simulink model "tutorial_switched_nets"  (R2020a)
settings: Solver=FixedStepAuto  StartTime=0.0  StopTime=options.T_train  FixedStep=options.dt  MaxStep=.2  RelTol=1e-3
model workspace (MAT data in the model file):
  PID_TRESH = 0.3
undefined symbols (not defined in the file or in its folder): DiscIntNeverNeededParam, options
libraries: neural x72, simulink x2
(part 3 of 3)

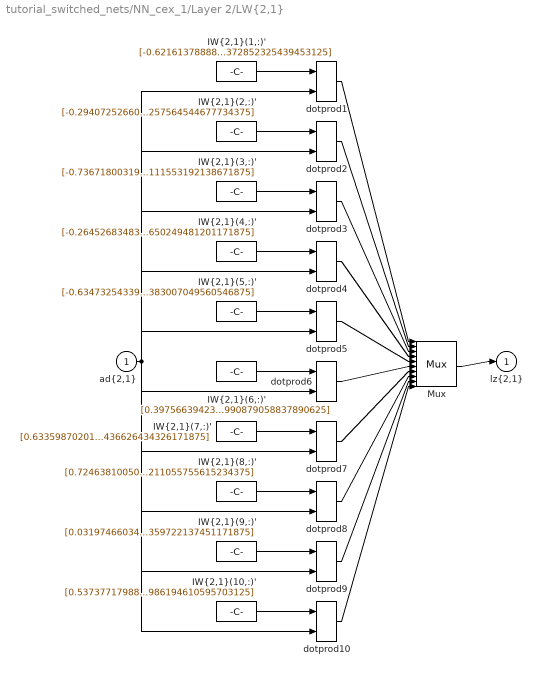
== system tutorial_switched_nets/NN_cex_1/Layer 2/LW{2,1} ==
  "ad{2,1}" : Inport  PortDimensions=20
      mask Display: e = 0.06;c1 = [120 230 180]/255;c2 = ([120 230 180]+0)/(256+128);c3 = ([120 230 180]+128)/(256+128);patch([0 1 1 0],[0 0 1 1],c1);patch([0 1 1 1-e 1-e 0+e],[0 0 1 1-e 0+e 0+e],c2);patch([0 0 1 1-e 0+e 0+e],[0 1 1 1-e 1-e 0+e],c3);plot([0 1 1 0 0],[0 0 1 1 0]);
  "IW{2,1}(1,:)'" : Constant  Value=[-0.62161378888258445041259392382926307618618011474609375;0.6148140198052960414543122169561684131622314453125;0.2096842513607183600132799483617418445646762847900390625;1.42295581141193760998930883943103253841400146484375;0.048162932797590825295674932249312405474483966827392578125;-0.329960676951758291597371908210334368050098419189453125;-0.243824039590348651262985413268324919044971466064453125;1.3156362099355323191929301174241118133068084716796875;0.65903370153445306467432374120107851922512054443359375;-0.1513918664553025872354652392459684051573276519775390625;-0.276008888794093854013311784001416526734828948974609375;0.476624595374437076689133618856430985033512115478515625;-0.7156998438142954110929849775857292115688323974609375;-0.350604636353502474577226166729815304279327392578125;0.359070507579784592433469470051932148635387420654296875;-0.088593367865525907145496375960647128522396087646484375;0.1682563802502727579035735061552259139716625213623046875;-0.157656333921617652915614371522678993642330169677734375;-0.082841065900426891221997038883273489773273468017578125;0.27502807794997086165977862037834711372852325439453125]
      mask Display: e = 0.06;c1 = [120 150 230]/255;c2 = ([120 150 230]+0)/383;c3 = ([120 150 230]+128)/383;patch([0 1 1 0],[0 0 1 1],c1);patch([0 1 1 1-e 1-e 0+e],[0 0 1 1-e 0+e 0+e],c2);patch([0 0 1 1-e 0+e 0+e],[0 1 1 1-e 1-e 0+e],c3);plot([0 1 1 0 0],[0 0 1 1 0]);disp('weights');
  "IW{2,1}(10,:)'" : Constant  Value=[0.53737717988913347166857192860334180295467376708984375;-0.54494791628668937111257264405139721930027008056640625;-0.327865563770393053655283210900961421430110931396484375;-0.2431502509493463082268505104366340674459934234619140625;-0.5506763502515099606426929312874563038349151611328125;0.2489329212039713412618624488459317944943904876708984375;0.2987323473001877172094964407733641564846038818359375;-0.37860104355034407408453489551902748644351959228515625;-0.523585007940606583787257477524690330028533935546875;0.25019101968781154443632885886472649872303009033203125;1.466831577856468005194301440496928989887237548828125;-0.68566639556574349168016624389565549790859222412109375;-0.51939265556673752666227983354474417865276336669921875;0.41255958958065652719682248061872087419033050537109375;-0.031873003307670851047550542034514364786446094512939453125;0.2298586870540712256971715987674542702734470367431640625;-0.2395025987128011346616318633095943368971347808837890625;0.39020251935073113624952156897052191197872161865234375;-0.14742684095521407794393553558620624244213104248046875;0.07941988847293768305490857528639025986194610595703125]
      mask Display: e = 0.06;c1 = [120 150 230]/255;c2 = ([120 150 230]+0)/383;c3 = ([120 150 230]+128)/383;patch([0 1 1 0],[0 0 1 1],c1);patch([0 1 1 1-e 1-e 0+e],[0 0 1 1-e 0+e 0+e],c2);patch([0 0 1 1-e 0+e 0+e],[0 1 1 1-e 1-e 0+e],c3);plot([0 1 1 0 0],[0 0 1 1 0]);disp('weights');
  "IW{2,1}(2,:)'" : Constant  Value=[-0.294072526609415518805690226145088672637939453125;1.524795289433424017033757991157472133636474609375;-0.11998592442710477590228634880986646749079227447509765625;0.88642225740235691677781915132072754204273223876953125;-1.13736511663246897541057478520087897777557373046875;0.56518577870423569731173074615071527659893035888671875;0.09829027065135671759055213669853401370346546173095703125;-1.0125569421073750131512269945233128964900970458984375;0.0165551729351459502026511216854487429372966289520263671875;0.82845463609548108951941003397223539650440216064453125;-0.9414506586527846554446341542643494904041290283203125;0.53562549536417181084146932334988377988338470458984375;-0.313691347770849782161661778445704840123653411865234375;0.47191275297145118816644071557675488293170928955078125;1.51617522055314868367759117973037064075469970703125;0.052764919032685243804881025653230608440935611724853515625;0.62185887535271133774728014032007195055484771728515625;0.0857756082959333643334076668907073326408863067626953125;0.25939285840393011550730761882732622325420379638671875;-0.224432553872412565709737464203499257564544677734375]
      mask Display: e = 0.06;c1 = [120 150 230]/255;c2 = ([120 150 230]+0)/383;c3 = ([120 150 230]+128)/383;patch([0 1 1 0],[0 0 1 1],c1);patch([0 1 1 1-e 1-e 0+e],[0 0 1 1-e 0+e 0+e],c2);patch([0 0 1 1-e 0+e 0+e],[0 1 1 1-e 1-e 0+e],c3);plot([0 1 1 0 0],[0 0 1 1 0]);disp('weights');
  "IW{2,1}(3,:)'" : Constant  Value=[-0.73671800319088820430124542326666414737701416015625;1.421314356877808382506600537453778088092803955078125;0.070753772050939911508748991764150559902191162109375;-0.56739678343006849647878198084072209894657135009765625;-0.85295856204789932686338715939200483262538909912109375;0.7386337240152494043599062933935783803462982177734375;0.0204718154347354776290135447425200254656374454498291015625;0.339184882494136863417821814437047578394412994384765625;-0.1881317420062826872850791914970614016056060791015625;-0.1339003061967665442200114966908586211502552032470703125;0.2394330914749966121579660693896585144102573394775390625;-0.6122315165013672011440348796895705163478851318359375;0.73620305612605718703633783661643974483013153076171875;0.38056001767816283187784165420453064143657684326171875;-0.1553003163997090096959396987585932947695255279541015625;0.0002292365914646561815548597706992950406856834888458251953125;0.0302889066986190315378113524502623477019369602203369140625;0.83805910127735006032168030287721194326877593994140625;0.1416795809112300352783364587594405747950077056884765625;-0.2543836837861146449313309858553111553192138671875]
      mask Display: e = 0.06;c1 = [120 150 230]/255;c2 = ([120 150 230]+0)/383;c3 = ([120 150 230]+128)/383;patch([0 1 1 0],[0 0 1 1],c1);patch([0 1 1 1-e 1-e 0+e],[0 0 1 1-e 0+e 0+e],c2);patch([0 0 1 1-e 0+e 0+e],[0 1 1 1-e 1-e 0+e],c3);plot([0 1 1 0 0],[0 0 1 1 0]);disp('weights');
  "IW{2,1}(4,:)'" : Constant  Value=[-0.264526834830059731640261588836438022553920745849609375;-0.84727523852972475015832287681405432522296905517578125;-0.443267493586528671389856981477350927889347076416015625;0.2034088335481475662280814731275313533842563629150390625;0.1795179798836086526581112821077113039791584014892578125;0.315091185795663253355058941451716236770153045654296875;-0.26441621089079669904009506353759206831455230712890625;0.167220214629539842832173235365189611911773681640625;0.4563687033643990531572853797115385532379150390625;0.49015080532649968336755819109384901821613311767578125;-0.554760108665810935946183235500939190387725830078125;1.386615644304538097486556580406613647937774658203125;-1.1832183710485491001662694543483667075634002685546875;-0.43202725012682130500962784935836680233478546142578125;-0.0781915813170765972017761669121682643890380859375;0.3670003065691587185170874363393522799015045166015625;-0.53144904234001433263046010324615053832530975341796875;0.09170220663540096239785270881839096546173095703125;0.307383388425944092947617036770679987967014312744140625;0.439267620633082500614108312220196239650249481201171875]
      mask Display: e = 0.06;c1 = [120 150 230]/255;c2 = ([120 150 230]+0)/383;c3 = ([120 150 230]+128)/383;patch([0 1 1 0],[0 0 1 1],c1);patch([0 1 1 1-e 1-e 0+e],[0 0 1 1-e 0+e 0+e],c2);patch([0 0 1 1-e 0+e 0+e],[0 1 1 1-e 1-e 0+e],c3);plot([0 1 1 0 0],[0 0 1 1 0]);disp('weights');
  "IW{2,1}(5,:)'" : Constant  Value=[-0.6347325433958459495187298671226017177104949951171875;0.5840875105178520154680654741241596639156341552734375;0.0185129059743385192271514227968509658239781856536865234375;0.0675491501162142904401974874417646788060665130615234375;-0.46347623111425739761415343309636227786540985107421875;0.5367073319569934941597466604434885084629058837890625;0.039973946687769622287955684214466600678861141204833984375;1.2723768169482980727735821346868760883808135986328125;-0.321897678504259820986277418342069722712039947509765625;-1.2345977915604351426992479900945909321308135986328125;0.492154948890192678323529662520741112530231475830078125;-0.401866198171296373775618349100113846361637115478515625;0.5440306452056520303273146055289544165134429931640625;-0.423235921326210462467543038656003773212432861328125;-0.987700420301937054290419837343506515026092529296875;-0.08534087543556227728469565363411675207316875457763671875;-0.452894783647901866263651982080773450434207916259765625;0.5243165524372823682597299921326339244842529296875;-0.029587533104634737568527924622685532085597515106201171875;-0.32642992677670956691571291230502538383007049560546875]
      mask Display: e = 0.06;c1 = [120 150 230]/255;c2 = ([120 150 230]+0)/383;c3 = ([120 150 230]+128)/383;patch([0 1 1 0],[0 0 1 1],c1);patch([0 1 1 1-e 1-e 0+e],[0 0 1 1-e 0+e 0+e],c2);patch([0 0 1 1-e 0+e 0+e],[0 1 1 1-e 1-e 0+e],c3);plot([0 1 1 0 0],[0 0 1 1 0]);disp('weights');
  "IW{2,1}(6,:)'" : Constant  Value=[0.397566394231556208271882724147872067987918853759765625;0.118656971446195746988649943887139670550823211669921875;0.69625463231482453974052759804180823266506195068359375;-0.31121163833689269306859159769373945891857147216796875;1.0288427889346694055205944096087478101253509521484375;0.04711099322052481053191286264336667954921722412109375;0.227017365001152437997689048643223941326141357421875;-0.63947472125603865844567508247564546763896942138671875;-0.9546246500317121519429974796366877853870391845703125;0.397656087069081898288658294404740445315837860107421875;-0.27414060996643530021543710972764529287815093994140625;0.98347019346885122814683199976570904254913330078125;-0.133233100428705231177417545040952973067760467529296875;0.1569545888976784098201022743523935787379741668701171875;0.2012949466256813424447358329416601918637752532958984375;0.025514049366083875469701780502873589284718036651611328125;0.36651890120507080172984615273890085518360137939453125;0.26586788949406037207978670267038978636264801025390625;0.08274920815151894093464335355747607536613941192626953125;0.1168075424937572714956246500150882638990879058837890625]
      mask Display: e = 0.06;c1 = [120 150 230]/255;c2 = ([120 150 230]+0)/383;c3 = ([120 150 230]+128)/383;patch([0 1 1 0],[0 0 1 1],c1);patch([0 1 1 1-e 1-e 0+e],[0 0 1 1-e 0+e 0+e],c2);patch([0 0 1 1-e 0+e 0+e],[0 1 1 1-e 1-e 0+e],c3);plot([0 1 1 0 0],[0 0 1 1 0]);disp('weights');
  "IW{2,1}(7,:)'" : Constant  Value=[0.63359870201613188722689073983929120004177093505859375;-0.75217613310241493440599924724665470421314239501953125;0.491516857564532616553520938396104611456394195556640625;-0.6773625406162206985527518554590642452239990234375;-0.001224365613213741765807895944817573763430118560791015625;-0.58448681772046129356823485068161971867084503173828125;0.059540306641803660003819942403424647636711597442626953125;-0.115626952076331945828968628120492212474346160888671875;-0.06648644816369979337888906911757658235728740692138671875;0.2083024172188013556361596556598669849336147308349609375;-1.1752443338289939589458299451507627964019775390625;0.94823387040849083096105687218368984758853912353515625;-0.55989320275143106275805848781601525843143463134765625;0.64316972044623732518431324933771975338459014892578125;0.11102419887687575705825793193071149289608001708984375;-0.1754052728964779206410895540102501399815082550048828125;0.1327921461547354742283033601779607124626636505126953125;0.451010051153054813966036817873828113079071044921875;0.155358442653016737278193204474519006907939910888671875;0.2008256774708993830369507804789463989436626434326171875]
      mask Display: e = 0.06;c1 = [120 150 230]/255;c2 = ([120 150 230]+0)/383;c3 = ([120 150 230]+128)/383;patch([0 1 1 0],[0 0 1 1],c1);patch([0 1 1 1-e 1-e 0+e],[0 0 1 1-e 0+e 0+e],c2);patch([0 0 1 1-e 0+e 0+e],[0 1 1 1-e 1-e 0+e],c3);plot([0 1 1 0 0],[0 0 1 1 0]);disp('weights');
  "IW{2,1}(8,:)'" : Constant  Value=[0.72463810050641763726986255278461612761020660400390625;-0.139255620023811366170463088565156795084476470947265625;0.51716746325489204583192304198746569454669952392578125;1.097636150854096825923988944850862026214599609375;0.198298618235760393258004796734894625842571258544921875;-0.4117787873029661316337524112896062433719635009765625;-0.46879268840439325405355930342921055853366851806640625;0.51323346242688583362934195974958129227161407470703125;0.5556688939482599121078010284691117703914642333984375;0.549414187854548430323120555840432643890380859375;-0.10906828231105573923098717159518855623900890350341796875;-0.3797789712912906789910039151436649262905120849609375;0.36503388255895519165505902492441236972808837890625;-0.2429637888408737733669795488822273910045623779296875;0.2426968650607133903829293331000371836125850677490234375;0.431316471447297844488133478080271743237972259521484375;0.415532661220290033821100905697676353156566619873046875;-0.266118340314429990822731042499071918427944183349609375;0.00523046920580453982008162228112269076518714427947998046875;-0.0801417836810785766399334306697710417211055755615234375]
      mask Display: e = 0.06;c1 = [120 150 230]/255;c2 = ([120 150 230]+0)/383;c3 = ([120 150 230]+128)/383;patch([0 1 1 0],[0 0 1 1],c1);patch([0 1 1 1-e 1-e 0+e],[0 0 1 1-e 0+e 0+e],c2);patch([0 0 1 1-e 0+e 0+e],[0 1 1 1-e 1-e 0+e],c3);plot([0 1 1 0 0],[0 0 1 1 0]);disp('weights');
  "IW{2,1}(9,:)'" : Constant  Value=[0.03197466034513803123662256666648318059742450714111328125;0.425385771276686364128494233227684162557125091552734375;-0.5080832249196844951910634335945360362529754638671875;0.348444613423557758569160114348051138222217559814453125;0.03716218422520345399107100092805922031402587890625;0.1357216337531434169338950823657796718180179595947265625;-0.226513260772801483522442822504672221839427947998046875;-0.6007362594124796562056189941358752548694610595703125;0.9257584615124134774788444701698608696460723876953125;-0.81075337318190265900597069048671983182430267333984375;0.268184943287032739878128495547571219503879547119140625;0.51508871689384927439192551901214756071567535400390625;-0.024683914809465405670874105226175743155181407928466796875;0.258724376998405281025128488181508146226406097412109375;0.16768030786232535067625804003910161554813385009765625;0.340860503983454410370512732697534374892711639404296875;0.313071032007370131378110045261564664542675018310546875;0.81011682839776921749574967179796658456325531005859375;-0.00948404390577326471267749496973920031450688838958740234375;0.450530228487466544162742820844869129359722137451171875]
      mask Display: e = 0.06;c1 = [120 150 230]/255;c2 = ([120 150 230]+0)/383;c3 = ([120 150 230]+128)/383;patch([0 1 1 0],[0 0 1 1],c1);patch([0 1 1 1-e 1-e 0+e],[0 0 1 1-e 0+e 0+e],c2);patch([0 0 1 1-e 0+e 0+e],[0 1 1 1-e 1-e 0+e],c3);plot([0 1 1 0 0],[0 0 1 1 0]);disp('weights');
  Mux : Mux  Inputs=10
      mask Display: e = 0.06;c1 = [120 150 230]/255;c2 = ([120 150 230]+0)/383;c3 = ([120 150 230]+128)/383;patch([0 1 1 0],[0 0 1 1],c1);patch([0 1 1 1-e 1-e 0+e],[0 0 1 1-e 0+e 0+e],c2);patch([0 0 1 1-e 0+e 0+e],[0 1 1 1-e 1-e 0+e],c3);plot([0 1 1 0 0],[0 0 1 1 0]);disp('Mux');
  dotprod{1..10} (10 alike) : neural/Weight Functions/dotprod
  "lz{2,1}" : Outport
      mask Display: e = 0.06;c1 = [120 230 180]/255;c2 = ([120 230 180]+0)/(256+128);c3 = ([120 230 180]+128)/(256+128);patch([0 1 1 0],[0 0 1 1],c1);patch([0 1 1 1-e 1-e 0+e],[0 0 1 1-e 0+e 0+e],c2);patch([0 0 1 1-e 0+e 0+e],[0 1 1 1-e 1-e 0+e],c3);plot([0 1 1 0 0],[0 0 1 1 0]);
  wires:
  "IW{2,1}(1,:)'"/1 -> dotprod1/1
  "ad{2,1}"/1 -> dotprod1/2, dotprod2/2, dotprod3/2, dotprod4/2, dotprod5/2, dotprod6/2, dotprod7/2, dotprod8/2, dotprod9/2, dotprod10/2
  dotprod1/1 -> Mux/1
  "IW{2,1}(2,:)'"/1 -> dotprod2/1
  dotprod2/1 -> Mux/2
  "IW{2,1}(3,:)'"/1 -> dotprod3/1
  dotprod3/1 -> Mux/3
  "IW{2,1}(4,:)'"/1 -> dotprod4/1
  dotprod4/1 -> Mux/4
  "IW{2,1}(5,:)'"/1 -> dotprod5/1
  dotprod5/1 -> Mux/5
  "IW{2,1}(6,:)'"/1 -> dotprod6/1
  dotprod6/1 -> Mux/6
  "IW{2,1}(7,:)'"/1 -> dotprod7/1
  dotprod7/1 -> Mux/7
  "IW{2,1}(8,:)'"/1 -> dotprod8/1
  dotprod8/1 -> Mux/8
  "IW{2,1}(9,:)'"/1 -> dotprod9/1
  dotprod9/1 -> Mux/9
  "IW{2,1}(10,:)'"/1 -> dotprod10/1
  dotprod10/1 -> Mux/10
  Mux/1 -> "lz{2,1}"/1

== system tutorial_switched_nets/NN_cex_1/Layer 3/Delays 1 ==
  "p{3}" : Inport  PortDimensions=10
      mask Display: e = 0.06;c1 = [120 230 180]/255;c2 = ([120 230 180]+0)/(256+128);c3 = ([120 230 180]+128)/(256+128);patch([0 1 1 0],[0 0 1 1],c1);patch([0 1 1 1-e 1-e 0+e],[0 0 1 1-e 0+e 0+e],c2);patch([0 0 1 1-e 0+e 0+e],[0 1 1 1-e 1-e 0+e],c3);plot([0 1 1 0 0],[0 0 1 1 0]);
  mux : Mux  Inputs=1
      mask Display: e = 0.06;c1 = [120 150 230]/255;c2 = ([120 150 230]+0)/383;c3 = ([120 150 230]+128)/383;patch([0 1 1 0],[0 0 1 1],c1);patch([0 1 1 1-e 1-e 0+e],[0 0 1 1-e 0+e 0+e],c2);patch([0 0 1 1-e 0+e 0+e],[0 1 1 1-e 1-e 0+e],c3);plot([0 1 1 0 0],[0 0 1 1 0]);disp('Mux')
  "pd{3,2}" : Outport
      mask Display: e = 0.06;c1 = [120 230 180]/255;c2 = ([120 230 180]+0)/(256+128);c3 = ([120 230 180]+128)/(256+128);patch([0 1 1 0],[0 0 1 1],c1);patch([0 1 1 1-e 1-e 0+e],[0 0 1 1-e 0+e 0+e],c2);patch([0 0 1 1-e 0+e 0+e],[0 1 1 1-e 1-e 0+e],c3);plot([0 1 1 0 0],[0 0 1 1 0]);
  wires:
  "p{3}"/1 -> mux/1
  mux/1 -> "pd{3,2}"/1

== system tutorial_switched_nets/NN_cex_1/Layer 3/LW{3,2} ==
  "ad{3,2}" : Inport  PortDimensions=10
      mask Display: e = 0.06;c1 = [120 230 180]/255;c2 = ([120 230 180]+0)/(256+128);c3 = ([120 230 180]+128)/(256+128);patch([0 1 1 0],[0 0 1 1],c1);patch([0 1 1 1-e 1-e 0+e],[0 0 1 1-e 0+e 0+e],c2);patch([0 0 1 1-e 0+e 0+e],[0 1 1 1-e 1-e 0+e],c3);plot([0 1 1 0 0],[0 0 1 1 0]);
  "IW{3,2}(1,:)'" : Constant  Value=[-0.7775350965639116207483994003268890082836151123046875;-1.231185247015106565271480576484464108943939208984375;-1.6559463436637604782930566216236911714076995849609375;-0.6677875744421724046873123370460234582424163818359375;-1.020790309808809137592788829351775348186492919921875;0.361898349044003975194527811254374682903289794921875;-1.765053684857026627952336639282293617725372314453125;1.0136047273471489038598747356445528566837310791015625;-0.11721466190464528700498902935578371398150920867919921875;0.538914883495946295255407676449976861476898193359375]
      mask Display: e = 0.06;c1 = [120 150 230]/255;c2 = ([120 150 230]+0)/383;c3 = ([120 150 230]+128)/383;patch([0 1 1 0],[0 0 1 1],c1);patch([0 1 1 1-e 1-e 0+e],[0 0 1 1-e 0+e 0+e],c2);patch([0 0 1 1-e 0+e 0+e],[0 1 1 1-e 1-e 0+e],c3);plot([0 1 1 0 0],[0 0 1 1 0]);disp('weights');
  Mux : Mux  Inputs=1
      mask Display: e = 0.06;c1 = [120 150 230]/255;c2 = ([120 150 230]+0)/383;c3 = ([120 150 230]+128)/383;patch([0 1 1 0],[0 0 1 1],c1);patch([0 1 1 1-e 1-e 0+e],[0 0 1 1-e 0+e 0+e],c2);patch([0 0 1 1-e 0+e 0+e],[0 1 1 1-e 1-e 0+e],c3);plot([0 1 1 0 0],[0 0 1 1 0]);disp('Mux');
  dotprod1 : neural/Weight Functions/dotprod
  "lz{3,2}" : Outport
      mask Display: e = 0.06;c1 = [120 230 180]/255;c2 = ([120 230 180]+0)/(256+128);c3 = ([120 230 180]+128)/(256+128);patch([0 1 1 0],[0 0 1 1],c1);patch([0 1 1 1-e 1-e 0+e],[0 0 1 1-e 0+e 0+e],c2);patch([0 0 1 1-e 0+e 0+e],[0 1 1 1-e 1-e 0+e],c3);plot([0 1 1 0 0],[0 0 1 1 0]);
  wires:
  "IW{3,2}(1,:)'"/1 -> dotprod1/1
  "ad{3,2}"/1 -> dotprod1/2
  dotprod1/1 -> Mux/1
  Mux/1 -> "lz{3,2}"/1

== stateflow chart tutorial_switched_nets/SwitchingController ==
  state STEADY
    entry: u = 0;
  state P
    du:
    u = p_control(e);
    state u = p_control(e) [function]
  state PID
    du:
    u = pid_control(e);
    state u = pid_control(e) [function]
  (default) -> STEADY
  STEADY -> P : [e > 0.01]
  P -> PID : [e < PID_TRESH]
  data: e function_input; u function_output; e function_input; u function_output; e input; u output double; PID output boolean; PID_TRESH parameter; P output boolean
